simulink model "model"  (R2015a)
settings: Solver=ode4  StartTime=0.0  StopTime=1000  FixedStep=0.01  RelTol=1e-3
values from neighbouring files (symbols this model uses):
  KD = Td * k    [get_IND.m]    (also in sterowanie.m = 0)
  KI = k / Ti    [get_IND.m]    (also in sterowanie.m = 0)
  KP = k    [get_IND.m]    (also in sterowanie.m = 5.35)
libraries: simulink x1
settings Model: Creator=pingwin  LastModifiedBy=pingwin

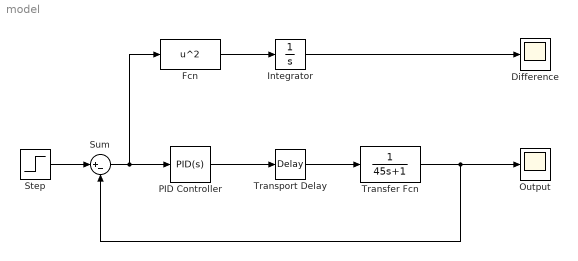
== system model ==
  Difference : Scope
      settings: SaveName=difference  MaxDataPoints=50000000  SampleInput=on
  Fcn : Fcn  Expr=u^2
  Integrator : Integrator
  Output : Scope
      settings: YMin=-8  YMax=9  SaveName=output  MaxDataPoints=50000000
  PID Controller : simulink/Continuous/PID Controller  Controller=PID  TimeDomain=Continuous-time  SampleTime=-1  IntegratorMethod=Forward Euler  FilterMethod=Forward Euler  Form=Parallel  UseFilter=on  ControllerParametersSource=internal  P=KP  I=KI  D=KD  N=100  InitialConditionSource=internal  InitialConditionForIntegrator=0  InitialConditionForFilter=0  ExternalReset=none  LimitOutput=off  UpperSaturationLimit=inf  LowerSaturationLimit=-inf  LinearizeAsGain=on  AntiWindupMode=none  Kb=1  TrackingMode=off  Kt=1  PParamMin=[]  PParamMax=[]  IParamMin=[]  IParamMax=[]  DParamMin=[]  DParamMax=[]  NParamMin=[]  NParamMax=[]  KbParamMin=[]  KbParamMax=[]  KtParamMin=[]  KtParamMax=[]  POutMin=[]  POutMax=[]  IOutMin=[]  IOutMax=[]  DOutMin=[]  DOutMax=[]  NOutMin=[]  NOutMax=[]  KbOutMin=[]  KbOutMax=[]  KtOutMin=[]  KtOutMax=[]  IntegratorOutMin=[]  IntegratorOutMax=[]  FilterOutMin=[]  FilterOutMax=[]  SumOutMin=[]  SumOutMax=[]  SumI1OutMin=[]  SumI1OutMax=[]  SumI2OutMin=[]  SumI2OutMax=[]  SumI3OutMin=[]  SumI3OutMax=[]  SumDOutMin=[]  SumDOutMax=[]  SaturationOutMin=[]  SaturationOutMax=[]  IntegratorContinuousStateAttributes=''  IntegratorStateMustResolveToSignalObject=off  IntegratorRTWStateStorageClass=Auto  FilterContinuousStateAttributes=''  FilterStateMustResolveToSignalObject=off  FilterRTWStateStorageClass=Auto  DifferentiatorICPrevScaledInput=0  DifferentiatorOutMin=[]  DifferentiatorOutMax=[]
  Step : Step  Time=0  SampleTime=0
  Sum : Sum  Inputs=|+-
  Transfer Fcn : TransferFcn  Denominator=[45 1]
  Transport Delay : TransportDelay  DelayTime=15  BufferSize=2048
  wires:
  Step/1 -> Sum/1
  Sum/1 -> Fcn/1, PID Controller/1
  PID Controller/1 -> Transport Delay/1
  Transport Delay/1 -> Transfer Fcn/1
  Transfer Fcn/1 -> Output/1, Sum/2
  Fcn/1 -> Integrator/1
  Integrator/1 -> Difference/1
